simulink model "designing"  (R2013a)
settings: Solver=ode45  StartTime=0.0  StopTime=10.0  RelTol=1e-3
settings Model: Creator=Administrator  LastModifiedBy=Administrator

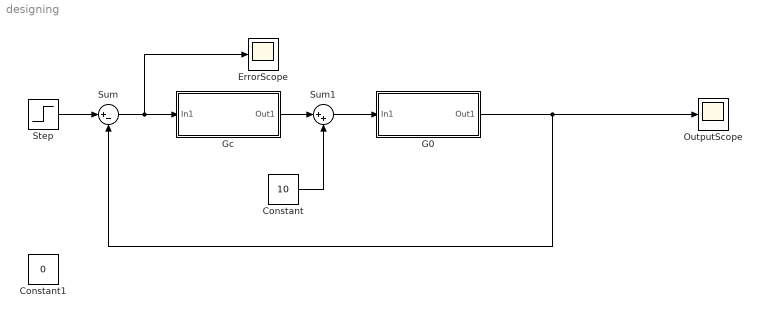
== system designing ==
  Constant : Constant  Value=10
  Constant1 : Constant  Value=0
  ErrorScope : Scope
  G0 : Subsystem
  Gc : Subsystem
  OutputScope : Scope
  Step : Step  SampleTime=0
  Sum : Sum  Inputs=|+-
  Sum1 : Sum  Inputs=|++
  wires:
  G0/1(Out1) -> OutputScope/1, Sum/2
  Sum/1 -> Gc/1(In1), ErrorScope/1
  Gc/1(Out1) -> Sum1/1
  Constant/1 -> Sum1/2
  Sum1/1 -> G0/1(In1)
  Step/1 -> Sum/1

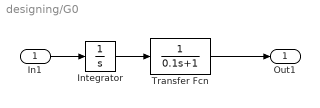
== system designing/G0 ==
  In1 : Inport
  Integrator : Integrator
  Transfer Fcn : TransferFcn  Denominator=[0.1 1]
  Out1 : Outport
  wires:
  In1/1 -> Integrator/1
  Integrator/1 -> Transfer Fcn/1
  Transfer Fcn/1 -> Out1/1

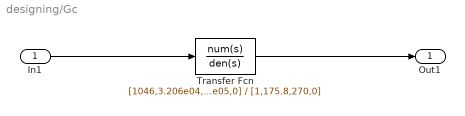
== system designing/Gc ==
  In1 : Inport
  Transfer Fcn : TransferFcn  Numerator=[1046,3.206e04,2.16e05,0]  Denominator=[1,175.8,270,0]
  Out1 : Outport
  wires:
  In1/1 -> Transfer Fcn/1
  Transfer Fcn/1 -> Out1/1
